simulink model "sfcndemo_simomex"  (Simulink 6.0)
settings: Solver=ode5  StartTime=0.0  StopTime=20  RelTol=1e-3
settings Model: Creator=The MathWorks Inc.  LastModifiedBy=batserve  ExtModeTrigMode=oneshot  ExtModeArmWhenConnect=off  ExtModeAutoUpdateStatusClock=off
settings DataIOCC: LimitDataPoints=off
settings OptimizationCC: BooleanDataType=off
settings DebuggingCC: CheckExecutionContextPreStartOutputMsg=on  CheckExecutionContextRuntimeOutputMsg=on  SolverPrmCheckMsg=none
settings HardwareCC: TargetUnknown=on

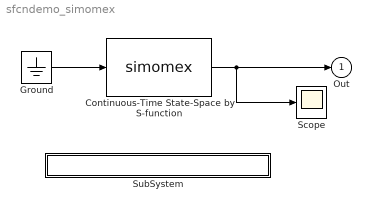
== system sfcndemo_simomex ==
  Continuous-Time State-Space by S-function : S-Function  FunctionName=simomex
      mask Type: S-function: simomex
      mask Description: This is a S-function block which has single-input and two output state-space system.
      mask Display: disp('dx/dt = A*X + B*U\nY      = C*X + D*U');
  Ground : Ground
  Scope : Scope
  SubSystem : Subsystem  PropExecContextAcrossSSBoundary=on
      settings: OpenFcn=edit(fullfile(matlabroot,'simulink','src','simomex.c'))
      mask Display: disp('matlabroot\simulink\src\simomex.c');
  Out : Outport  InitialOutput=0
  wires:
  Ground/1 -> Continuous-Time State-Space by S-function/1
  Continuous-Time State-Space by S-function/1 -> Out/1, Scope/1

== system sfcndemo_simomex/SubSystem ==
